simulink model "i_v_flux_of_memristor"  (Simulink 6.6)
settings: Solver=ode45  StartTime=0.0  StopTime=50  FixedStep=0.01  MaxStep=0.01  RelTol=1e-3
libraries: simulink x2
settings Model: Creator=Thang M. Hoang  LastModifiedBy=Thang M. Hoang  BufferReuse=off
settings DataIOCC: SaveOutput=off  SaveTime=off
settings OptimizationCC: ConditionallyExecuteInputs=off  InlineParams=on  InlineInvariantSignals=on  OptimizeBlockIOStorage=off  BufferReuse=off  ExpressionFolding=off  LocalBlockOutputs=off
settings DebuggingCC: SignalResolutionControl=TryResolveAllWithWarning  MultiTaskDSMMsg=warning  MultiTaskCondExecSysMsg=none  StrictBusMsg=None
settings RTWCC: SystemTargetFile=rtwin.tlc  TemplateMakefile=rtwin.tmf  Description=Real-Time Windows Target  ProcessScript=rtwin_make_rtw_hook  IncludeERTFirstTime=on
settings RTWinTargetCC: TargetFcnLib=ansi_tfl_tmw.mat  GenFloatMathFcnCalls=ANSI_C  ModelReferenceCompliant=off  PortableWordSizes=off  CCOptimize=on

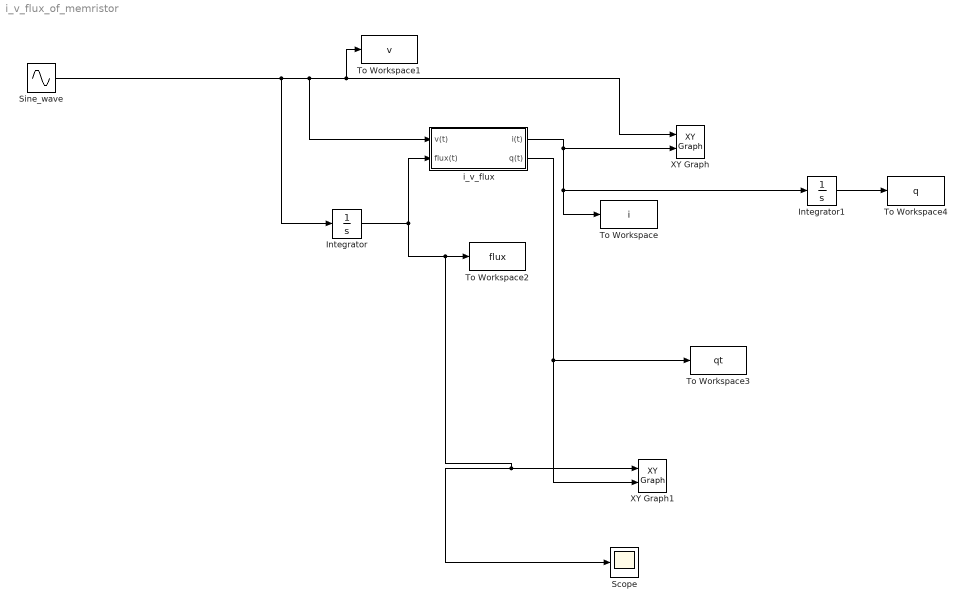
== system i_v_flux_of_memristor ==
  Integrator : Integrator
  Integrator1 : Integrator
  Scope : Scope
      settings: YMin=5.55112e-017  YMax=2  MaxDataPoints=50000
  Sine_wave : Sin  Amplitude=1.000000000000000000000000000000  Bias=0.000000000000000000000000000000  Frequency=5.000000000000000000000000000000  Phase=0.000000000000000000000000000000  SampleTime=0
  To Workspace : ToWorkspace  VariableName=i  SampleTime=-1  SaveFormat=Array
  To Workspace1 : ToWorkspace  VariableName=v  SampleTime=-1  SaveFormat=Array
  To Workspace2 : ToWorkspace  VariableName=flux  SampleTime=-1  SaveFormat=Array
  To Workspace3 : ToWorkspace  VariableName=qt  SampleTime=-1  SaveFormat=Array
  To Workspace4 : ToWorkspace  VariableName=q  SampleTime=-1  SaveFormat=Array
  XY Graph : simulink/Sinks/XY Graph  SystemSampleTime=-1  xmin=-1  xmax=1  ymin=-0.0002  ymax=0.0002  st=-1
  XY Graph1 : simulink/Sinks/XY Graph  SystemSampleTime=-1  xmin=0  xmax=2.5  ymin=-0.002  ymax=0.002  st=-1
  i_v_flux : Subsystem
  wires:
  Sine_wave/1 -> i_v_flux/1(v(t)), To Workspace1/1, XY Graph/1, Integrator/1
  i_v_flux/1(i(t)) -> XY Graph/2, To Workspace/1, Integrator1/1
  i_v_flux/2(q(t)) -> To Workspace3/1, XY Graph1/2
  Integrator/1 -> i_v_flux/2(flux(t)), To Workspace2/1, Scope/1, XY Graph1/1
  Integrator1/1 -> To Workspace4/1

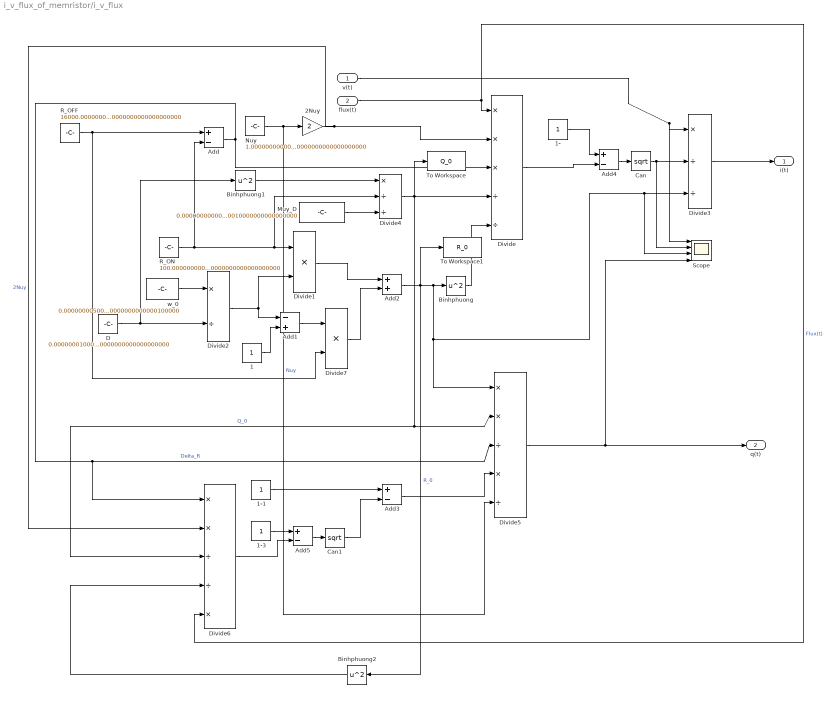
== system i_v_flux_of_memristor/i_v_flux ==
  v(t) : Inport
  flux(t) : Inport  Port=2
  1 : Constant
  1- : Constant
  1-1 : Constant
  1-3 : Constant
  2Nuy : Gain  Gain=2
  Add{,3..5} (4 alike) : Sum  Inputs=+-  OutScaling=2^-10
  Add1 : Sum  Inputs=-+  OutScaling=2^-10
  Add2 : Sum  OutScaling=2^-10
  Binhphuong : Math  Operator=square  SaturateOnIntegerOverflow=on
  Binhphuong1 : Math  Operator=square  SaturateOnIntegerOverflow=on
  Binhphuong2 : Math  Orientation=left  Operator=square  SaturateOnIntegerOverflow=on
  Can : Math  Operator=sqrt  SaturateOnIntegerOverflow=on
  Can1 : Math  Operator=sqrt  SaturateOnIntegerOverflow=on
  D : Constant  Value=0.000000010000000000000000000000
  Divide : Product  Inputs=***//  OutScaling=2^-10
  Divide1 : Product  Inputs=**  OutScaling=2^-10
  Divide2 : Product  Inputs=*/  OutScaling=2^-10
  Divide3 : Product  Inputs=*//  OutScaling=2^-10
  Divide4 : Product  Inputs=*//  OutScaling=2^-10
  Divide5 : Product  Inputs=**/*/  OutScaling=2^-10
  Divide6 : Product  Inputs=**//*  OutScaling=2^-10
  Divide7 : Product  Inputs=**  OutScaling=2^-10
  Muy_D : Constant  Value=0.000000000000010000000000000000
  Nuy : Constant  Value=1.000000000000000000000000000000
  R_OFF : Constant  Value=16000.000000000000000000000000000000
  R_ON : Constant  Value=100.000000000000000000000000000000
  Scope : Scope  NumInputPorts=4
      settings: YMin=-1~-500~50.5~0  YMax=1~50~50.5~0.00016  MaxDataPoints=50000
  To Workspace : ToWorkspace  VariableName=Q_0  SampleTime=-1  SaveFormat=Array
  To Workspace1 : ToWorkspace  VariableName=R_0  SampleTime=-1  SaveFormat=Array
  w_0 : Constant  Value=0.000000005000000000000000100000
  i(t) : Outport
  q(t) : Outport  Port=2
  wires:
  R_ON/1 -> Add/2, Divide1/1, Divide4/2
  w_0/1 -> Divide2/1
  D/1 -> Divide2/2, Binhphuong1/1
  Divide2/1 -> Divide1/2, Add1/1
  1/1 -> Add1/2
  Divide1/1 -> Add2/1
  R_OFF/1 -> Add/1, Divide7/2
  Add2/1 -> Binhphuong/1, Divide3/3, Scope/3, Divide5/1, Binhphuong2/1, To Workspace1/1  "R_0"
  Nuy/1 -> 2Nuy/1, Divide5/5  "Nuy"
  flux(t)/1 -> Divide/1, Divide6/5  "Flux(t)"
  2Nuy/1 -> Divide/2, Divide6/2  "2Nuy"
  Add/1 -> Divide/3, Divide5/3, Divide6/1  "Delta_R"
  Divide4/1 -> Divide/4, To Workspace/1, Divide5/2, Divide6/3  "Q_0"
  Binhphuong/1 -> Divide/5
  Divide/1 -> Add4/2
  1-/1 -> Add4/1
  v(t)/1 -> Divide3/1, Scope/1
  Add4/1 -> Can/1
  Divide3/1 -> i(t)/1
  Binhphuong1/1 -> Divide4/1
  Muy_D/1 -> Divide4/3
  1-1/1 -> Add3/1
  Can1/1 -> Add3/2
  Binhphuong2/1 -> Divide6/4
  1-3/1 -> Add5/1
  Divide6/1 -> Add5/2
  Add5/1 -> Can1/1
  Add3/1 -> Divide5/4
  Divide5/1 -> q(t)/1, Scope/4
  Can/1 -> Divide3/2, Scope/2
  Add1/1 -> Divide7/1
  Divide7/1 -> Add2/2
